simulink subsystem "TMS"  (R2023b)
settings: Solver=VariableStepAuto  StartTime=0.0  StopTime=10.0  RelTol=1e-3
libraries: simulink x1
settings Model: Creator=rebek  LastModifiedBy=nickj

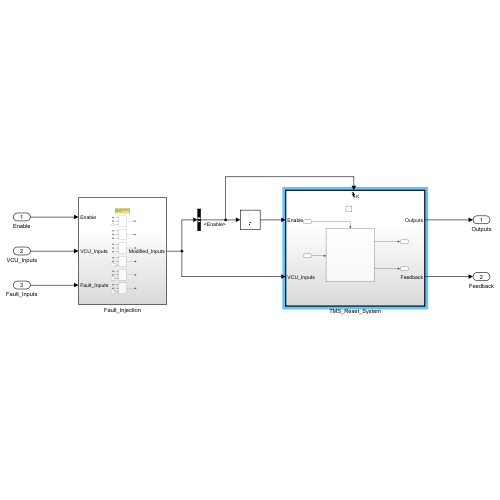
[thumbnail: Simulink's stored preview of the top-level diagram]
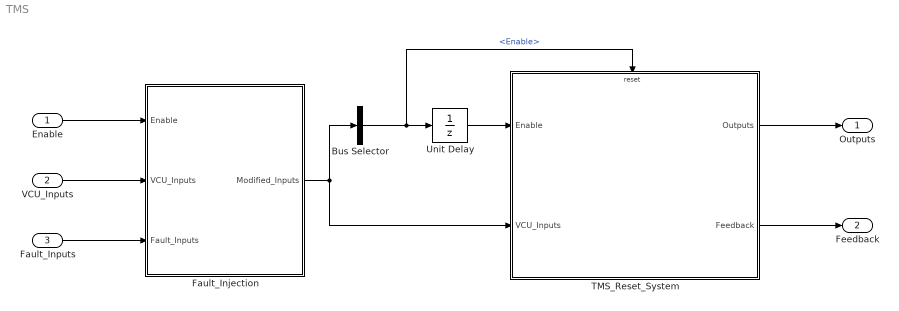
== system TMS ==
  Enable : Inport
  VCU_Inputs : Inport  Port=2
  Fault_Inputs : Inport  Port=3
  Bus Selector : BusSelector  OutputSignals=Enable
  Fault_Injection : Subsystem
  "TMS_Reset_System " : Subsystem  TreatAsAtomicUnit=on
  Unit Delay : UnitDelay  SampleTime=-1  HasFrameUpgradeWarning=on
  Outputs : Outport
  Feedback : Outport  Port=2
  wires:
  "TMS_Reset_System "/1(Outputs) -> Outputs/1
  "TMS_Reset_System "/2(Feedback) -> Feedback/1
  Fault_Injection/1(Modified_Inputs) -> "TMS_Reset_System "/2(VCU_Inputs), Bus Selector/1
  Unit Delay/1 -> "TMS_Reset_System "/1(Enable)
  Fault_Inputs/1 -> Fault_Injection/3(Fault_Inputs)
  VCU_Inputs/1 -> Fault_Injection/2(VCU_Inputs)
  Enable/1 -> Fault_Injection/1(Enable)
  Bus Selector/1 -> Unit Delay/1, "TMS_Reset_System "/Reset  "<Enable>"

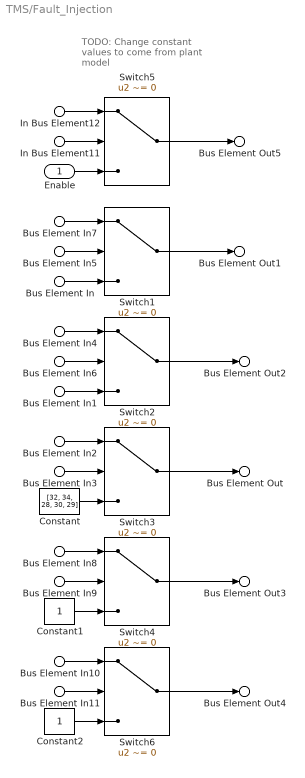
== system TMS/Fault_Injection ==
  note: TODO: Change constant values to come from plant model
  Enable : Inport
  Bus Element In : Inport  Port=2  PortName=VCU_Inputs  Element=TMS_Outputs.MC_Speed
  Bus Element In1 : Inport  Port=2  PortName=VCU_Inputs  Element=TMS_Outputs.Batt_Speed
  Bus Element In2 : Inport  Port=3  PortName=Fault_Inputs  Element=Temperatures
  Bus Element In3 : Inport  Port=3  PortName=Fault_Inputs  Element=Override_Temperatures
  Bus Element In10 : Inport  Port=3  PortName=Fault_Inputs  Element=MC_Flow_Rate
  Bus Element In9 : Inport  Port=3  PortName=Fault_Inputs  Element=Override_Batt_FR
  Bus Element In8 : Inport  Port=3  PortName=Fault_Inputs  Element=Batt_Flow_Rate
  Bus Element In11 : Inport  Port=3  PortName=Fault_Inputs  Element=Override_MC_FR
  Bus Element In7 : Inport  Port=3  PortName=Fault_Inputs  Element=MC_Speed
  Bus Element In5 : Inport  Port=3  PortName=Fault_Inputs  Element=Override_MC_Speed
  Bus Element In4 : Inport  Port=3  PortName=Fault_Inputs  Element=Batt_Speed
  Bus Element In6 : Inport  Port=3  PortName=Fault_Inputs  Element=Override_Batt_Speed
  In Bus Element12 : Inport  Port=3  PortName=Fault_Inputs  Element=TMS_EN
  In Bus Element11 : Inport  Port=3  PortName=Fault_Inputs  Element=Override_TMS_EN
  Constant : Constant  Value=[32, 34, 28, 30, 29]
  Constant1 : Constant
  Constant2 : Constant
  Switch{1..6} (6 alike) : Switch  Criteria=u2 ~= 0  SaturateOnIntegerOverflow=off  InputSameDT=off
  Bus Element Out : Outport  PortName=Modified_Inputs  Element=Temperatures
  Bus Element Out3 : Outport  PortName=Modified_Inputs  Element=Batt_Flow_Rate
  Bus Element Out4 : Outport  PortName=Modified_Inputs  Element=MC_Flow_Rate
  Bus Element Out1 : Outport  PortName=Modified_Inputs  Element=MC_Speed
  Bus Element Out2 : Outport  PortName=Modified_Inputs  Element=Batt_Speed
  Bus Element Out5 : Outport  PortName=Modified_Inputs  Element=Enable
  wires:
  Switch6/1 -> Bus Element Out4/1
  Switch4/1 -> Bus Element Out3/1
  Switch3/1 -> Bus Element Out/1
  Switch2/1 -> Bus Element Out2/1
  Switch1/1 -> Bus Element Out1/1
  Switch5/1 -> Bus Element Out5/1
  Constant/1 -> Switch3/3
  Bus Element In2/1 -> Switch3/1
  Bus Element In3/1 -> Switch3/2
  Bus Element In1/1 -> Switch2/3
  Bus Element In/1 -> Switch1/3
  Bus Element In6/1 -> Switch2/2
  Bus Element In4/1 -> Switch2/1
  Bus Element In5/1 -> Switch1/2
  Bus Element In7/1 -> Switch1/1
  Bus Element In9/1 -> Switch4/2
  Constant1/1 -> Switch4/3
  Bus Element In8/1 -> Switch4/1
  Bus Element In10/1 -> Switch6/1
  Constant2/1 -> Switch6/3
  Bus Element In11/1 -> Switch6/2
  In Bus Element12/1 -> Switch5/1
  In Bus Element11/1 -> Switch5/2
  Enable/1 -> Switch5/3

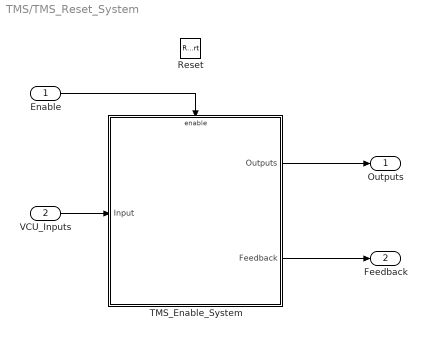
== system TMS/TMS_Reset_System  ==
  Enable : Inport
  VCU_Inputs : Inport  Port=2
  Reset : ResetPort  DisableCoverage=on  ResetTriggerType=falling
  "TMS_Enable_System " : Subsystem  TreatAsAtomicUnit=on
  Outputs : Outport
  Feedback : Outport  Port=2
  wires:
  VCU_Inputs/1 -> "TMS_Enable_System "/1(Input)
  "TMS_Enable_System "/2(Feedback) -> Feedback/1
  "TMS_Enable_System "/1(Outputs) -> Outputs/1
  Enable/1 -> "TMS_Enable_System "/Enable

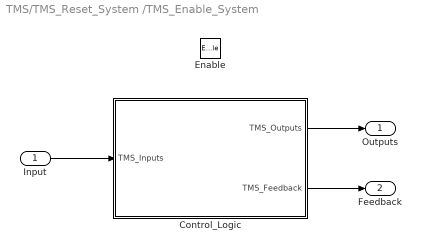
== system TMS/TMS_Reset_System /TMS_Enable_System  ==
  Input : Inport
  Enable : EnablePort  StatesWhenEnabling=reset
  Control_Logic : Subsystem
  Outputs : Outport
  Feedback : Outport  Port=2
  wires:
  Input/1 -> Control_Logic/1(TMS_Inputs)
  Control_Logic/2(TMS_Feedback) -> Feedback/1
  Control_Logic/1(TMS_Outputs) -> Outputs/1

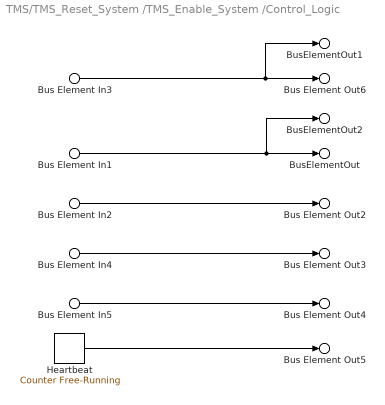
== system TMS/TMS_Reset_System /TMS_Enable_System /Control_Logic ==
  Bus Element In2 : Inport  PortName=TMS_Inputs  Element=Temperatures
  Bus Element In4 : Inport  PortName=TMS_Inputs  Element=Batt_Flow_Rate
  Bus Element In5 : Inport  PortName=TMS_Inputs  Element=MC_Flow_Rate
  Bus Element In3 : Inport  PortName=TMS_Inputs  Element=Batt_Speed
  Bus Element In1 : Inport  PortName=TMS_Inputs  Element=MC_Speed
  Heartbeat : simulink/Sources/Counter Free-Running  NumBits=32  tsamp=-1
  Bus Element Out6 : Outport  PortName=TMS_Outputs  Element=Batt_Speed_Out
  BusElementOut : Outport  PortName=TMS_Outputs  Element=MC_Speed_Out
  Bus Element Out3 : Outport  Port=2  PortName=TMS_Feedback  Element=Batt_Flow_Rate
  Bus Element Out4 : Outport  Port=2  PortName=TMS_Feedback  Element=MC_Flow_Rate
  Bus Element Out5 : Outport  Port=2  PortName=TMS_Feedback  Element=TMS_Heartbeat
  Bus Element Out2 : Outport  Port=2  PortName=TMS_Feedback  Element=Temperatures
  BusElementOut1 : Outport  Port=2  PortName=TMS_Feedback  Element=Batt_Speed_Out
  BusElementOut2 : Outport  Port=2  PortName=TMS_Feedback  Element=MC_Speed_Out
  wires:
  Bus Element In2/1 -> Bus Element Out2/1
  Bus Element In5/1 -> Bus Element Out4/1
  Bus Element In4/1 -> Bus Element Out3/1
  Heartbeat/1 -> Bus Element Out5/1
  Bus Element In3/1 -> Bus Element Out6/1, BusElementOut1/1
  Bus Element In1/1 -> BusElementOut2/1, BusElementOut/1
